simulink model "HMG_1DG1_Test_Cases"  (R2015b)
settings: Solver=ode23tb  StartTime=0.0  StopTime=.3  RelTol=1e-3
undefined symbols (not defined in the file or in its folder): tac, tdc, tdc1
libraries: powerlib x46, powerlib_meascontrol x14, simulink_extras x10, simulink x4
settings Model: Creator=Masoud  LastModifiedBy=Masoud

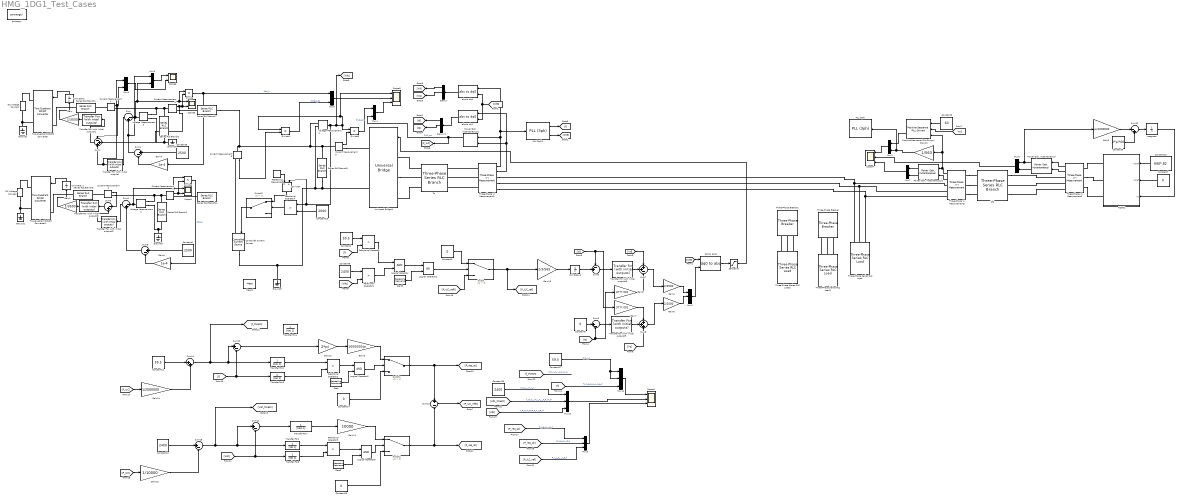
== system HMG_1DG1_Test_Cases ==
  ACDG1 : Subsystem
  Constant1 : Constant  Value=59.5
  Constant10 : Constant  Value=690*.82
  Constant11 : Constant  Value=59.5
  Constant12 : Constant  Value=2400
  Constant{4,6..7,13..14} (5 alike) : Constant  Value=0
  Constant15 : Constant  Value=2000
  Constant16 : Constant  Value=2400
  Constant17 : Constant  Value=59.5
  Constant2 : Constant  Value=2500
  Constant3 : Constant  Value=60
  Constant5 : Constant  Value=2*pi*60
  Constant8 : Constant  Value=2500
  Constant9 : Constant  Value=2400
  Controlled Current Source : powerlib/Electrical Sources/Controlled Current Source  Initialize=on  Source_Type=AC  Amplitude=0  Phase=0  Frequency=0  Measurements=None
  Current Measurement{1..6} (6 alike) : powerlib/Measurements/Current Measurement  PhasorSimulation=off  OutputType=Complex  PSBequivalent=0
  DC Voltage Source1 : powerlib/Electrical Sources/DC Voltage Source  Amplitude=3500  Measurements=None
  DC Voltage Source2 : powerlib/Electrical Sources/DC Voltage Source  Amplitude=3500  Measurements=None
  Demux : Demux  Outputs=3
  Demux1 : Demux  Outputs=3
  Divide{,1..3} (4 alike) : Product  Inputs=**
  Divide4 : Product  Inputs=*/
  Gain : Gain  Gain=1/3500
  Gain1 : Gain  Gain=1/3500
  Gain10 : Gain  Gain=1/563
  Gain11 : Gain  Gain=10000
  Gain12 : Gain  Gain=2*pi
  Gain13 : Gain  Gain=2/3/565
  Gain14 : Gain  Gain=1/2000000
  Gain15 : Gain  Gain=1/10000
  Gain2 : Gain  Gain=2/2500
  Gain3 : Gain  Gain=pi/1000000
  Gain4 : Gain  Gain=1e-4
  Gain5 : Gain  Gain=377*.001
  Gain6 : Gain  Gain=2/2500
  Gain7 : Gain  Gain=377*.001
  Gain8 : Gain  Gain=1e-4
  Gain9 : Gain  Gain=1000000/pi
  Ground{1..5} (5 alike) : powerlib/Elements/Ground  LConnTagsString=a
  Integrator : Integrator
  Logical Operator : Logic  AllPortsSameDT=off  OutDataTypeStr=boolean
  Logical Operator1 : Logic  Operator=OR  AllPortsSameDT=off  OutDataTypeStr=boolean
  Logical Operator2 : Logic  AllPortsSameDT=off  OutDataTypeStr=boolean
  Logical Operator3 : Logic  AllPortsSameDT=off  OutDataTypeStr=boolean
  Mean1 : powerlib_meascontrol/Measurements/Mean  Freq=10  Vinit=0  Ts=0
  Mux{1,4,6..9} (6 alike) : Mux  Inputs=2
  Mux{2..3,5,10..11} (5 alike) : Mux  Inputs=3
  PLL (3ph) : powerlib_meascontrol/PLL/PLL (3ph)  Fmin=45  Par_Init=[0, 60]  ParK=[180, 3200, 1]  TcD=1e-4  MaxRateChangeFreq=12  FilterCutOffFreq=25  Ts=0  AGC=on
  PLL (3ph)1 : powerlib_meascontrol/PLL/PLL (3ph)  Fmin=45  Par_Init=[0, 60]  ParK=[180, 3200, 1]  TcD=1e-4  MaxRateChangeFreq=12  FilterCutOffFreq=25  Ts=0  AGC=on
  Positive-Sequence (PLL-Driven) : powerlib_meascontrol/Measurements/Positive-Sequence (PLL-Driven)  Finit=60  Fmin=45  InInit=[1, 0]  Ts=0
  "Power (3ph, Instantaneous)" : powerlib_meascontrol/Measurements/Power (3ph, Instantaneous)
  "Power (3ph, Instantaneous)1" : powerlib_meascontrol/Measurements/Power (3ph, Instantaneous)
  "Power (3ph, Instantaneous)2" : powerlib_meascontrol/Measurements/Power (3ph, Instantaneous)
  Relational Operator{,1..4} (5 alike) : RelationalOperator  Operator=>  OutDataTypeStr=boolean
  Repeating Sequence3 : simulink/Sources/Repeating Sequence  rep_seq_t=[0 .1 .1001 .2 .2001 10]  rep_seq_y=1e3*[500 500 1800 1800 500 500]
  Saturation : Saturate  UpperLimit=1  LowerLimit=-1
  Scope1 : Scope  NumInputPorts=2
  Scope2 : Scope  NumInputPorts=3
  Scope3 : Scope  NumInputPorts=2
  Scope4 : Scope  NumInputPorts=3
  Scope5 : Scope  NumInputPorts=3
  Scope6 : Scope  NumInputPorts=2
  Series RLC Branch1 : powerlib/Elements/Series RLC Branch  LConnTagsString=__new0  RConnTagsString=__new0  BranchType=RL  Resistance=.05  Inductance=1e-3  SetiL0=off  InitialCurrent=0  Capacitance=1e-6  Setx0=off  InitialVoltage=0  Measurements=None
  Series RLC Branch2 : powerlib/Elements/Series RLC Branch  LConnTagsString=__new0  RConnTagsString=__new0  BranchType=C  Resistance=.05  Inductance=1e-3  SetiL0=off  InitialCurrent=0  Capacitance=4700e-6  Setx0=off  InitialVoltage=0  Measurements=None
  Series RLC Branch3 : powerlib/Elements/Series RLC Branch  LConnTagsString=__new0  RConnTagsString=__new0  BranchType=RL  Resistance=.05  Inductance=1e-3  SetiL0=off  InitialCurrent=0  Capacitance=1e-6  Setx0=off  InitialVoltage=0  Measurements=None
  Series RLC Branch4 : powerlib/Elements/Series RLC Branch  LConnTagsString=__new0  RConnTagsString=__new0  BranchType=C  Resistance=.05  Inductance=1e-3  SetiL0=off  InitialCurrent=0  Capacitance=4700e-6  Setx0=off  InitialVoltage=0  Measurements=None
  Series RLC Branch6 : powerlib/Elements/Series RLC Branch  LConnTagsString=__new0  RConnTagsString=__new0  BranchType=R  Resistance=.01  Inductance=1e-3  SetiL0=off  InitialCurrent=0  Capacitance=1e-6  Setx0=off  InitialVoltage=0  Measurements=None
  Series RLC Branch7 : powerlib/Elements/Series RLC Branch  LConnTagsString=__new0  RConnTagsString=__new0  BranchType=R  Resistance=.01  Inductance=1e-3  SetiL0=off  InitialCurrent=0  Capacitance=1e-6  Setx0=off  InitialVoltage=0  Measurements=None
  Series RLC Branch8 : powerlib/Elements/Series RLC Branch  LConnTagsString=__new0  RConnTagsString=__new0  BranchType=C  Resistance=.05  Inductance=1e-3  SetiL0=off  InitialCurrent=0  Capacitance=4700e-6  Setx0=on  InitialVoltage=2500  Measurements=None
  Start : simulink/Sources/Repeating Sequence  rep_seq_t=[0 .1 .1001 10]  rep_seq_y=[0 0 1 1]
  Start2 : simulink/Sources/Repeating Sequence  rep_seq_t=[0 .1 .1001 10]  rep_seq_y=[0 0 1 1]
  Start3 : simulink/Sources/Repeating Sequence  rep_seq_t=[0 .1 .1001 10]  rep_seq_y=[1 1 0 0]
  Sum{,2..3,12} (4 alike) : Sum  Inputs=|-+
  Sum1 : Sum  Inputs=-++
  Sum{4..5,9..11,15} (6 alike) : Sum  Inputs=|+-
  Sum13 : Sum  Inputs=+-
  Sum14 : Sum  Inputs=|++
  Sum6 : Sum  Inputs=-+|
  Sum7 : Sum  Inputs=++-
  Sum8 : Sum  Inputs=+++
  Switch{,1..3} (4 alike) : Switch  Criteria=u2 > Threshold  Threshold=.5
  Three-Phase Series RLC Load : powerlib/Elements/Three-Phase Series RLC Load  LConnTagsString=A|B|C  Configuration=Y (grounded)  NominalVoltage=690  Vabc=[1e3 1e3 1e3]  Vabcp=[1e3 1e3 1e3]  NominalFrequency=60  UnbalancedPower=off  ActivePower=100e3  InductivePower=0  CapacitivePower=0  Pabc=[10e3 9e3 11e3]  QLabc=[100 90 110]  QCabc=[100 90 110]  Pabcp=[10e3 9e3 11e3]  QLabcp=[100 90 110]  QCabcp=[100 90 110]  Measurements=None  LoadType=constant I
  Three-Phase Series RLC Load1 : powerlib/Elements/Three-Phase Series RLC Load  LConnTagsString=A|B|C  Configuration=Y (grounded)  NominalVoltage=690  Vabc=[1e3 1e3 1e3]  Vabcp=[1e3 1e3 1e3]  NominalFrequency=60  UnbalancedPower=off  ActivePower=1200e3  InductivePower=0  CapacitivePower=0  Pabc=[10e3 9e3 11e3]  QLabc=[100 90 110]  QCabc=[100 90 110]  Pabcp=[10e3 9e3 11e3]  QLabcp=[100 90 110]  QCabcp=[100 90 110]  Measurements=None  LoadType=constant I
  Three-Phase Series RLC Load2 : powerlib/Elements/Three-Phase Series RLC Load  LConnTagsString=A|B|C  Configuration=Y (grounded)  NominalVoltage=690  Vabc=[1e3 1e3 1e3]  Vabcp=[1e3 1e3 1e3]  NominalFrequency=60  UnbalancedPower=off  ActivePower=500e3  InductivePower=0  CapacitivePower=0  Pabc=[10e3 9e3 11e3]  QLabc=[100 90 110]  QCabc=[100 90 110]  Pabcp=[10e3 9e3 11e3]  QLabcp=[100 90 110]  QCabcp=[100 90 110]  Measurements=None  LoadType=constant I
  Three-Phase V-I Measurement1 : powerlib/Measurements/Three-Phase V-I Measurement  VoltageMeasurement=phase-to-ground  SetLabelV=off  LabelV=Vabc  Vpu=off  VpuLL=off  CurrentMeasurement=yes  SetLabelI=off  LabelI=Iabc  Ipu=off  Pbase=100e6  Vbase=500e3  OutputType=Complex  PhasorSimulation=off  PSBequivalent=0
  Three-Phase V-I Measurement2 : powerlib/Measurements/Three-Phase V-I Measurement  VoltageMeasurement=phase-to-ground  SetLabelV=off  LabelV=Vabc  Vpu=off  VpuLL=off  CurrentMeasurement=yes  SetLabelI=off  LabelI=Iabc  Ipu=off  Pbase=100e6  Vbase=500e3  OutputType=Complex  PhasorSimulation=off  PSBequivalent=0
  Three-Phase V-I Measurement5 : powerlib/Measurements/Three-Phase V-I Measurement  VoltageMeasurement=phase-to-ground  SetLabelV=off  LabelV=Vabc  Vpu=off  VpuLL=off  CurrentMeasurement=yes  SetLabelI=off  LabelI=Iabc  Ipu=off  Pbase=100e6  Vbase=500e3  OutputType=Complex  PhasorSimulation=off  PSBequivalent=0
  Three-Phase Breaker : powerlib/Elements/Three-Phase Breaker  InitialState=open  SwitchA=on  SwitchB=on  SwitchC=on  SwitchTimes=[.2 .6]  External=off  BreakerResistance=0.01  SnubberResistance=1e6  SnubberCapacitance=inf  Measurements=None
  Three-Phase Breaker1 : powerlib/Elements/Three-Phase Breaker  InitialState=open  SwitchA=on  SwitchB=on  SwitchC=on  SwitchTimes=[.4 .7]  External=off  BreakerResistance=0.01  SnubberResistance=1e6  SnubberCapacitance=inf  Measurements=None
  Transfer Fcn (with initial outputs) : simulink_extras/Additional Linear/Transfer Fcn (with initial outputs)  N=[8 1]  D=[1 0]  Y0=.5  U0=0
  Transfer Fcn (with initial outputs)1 : simulink_extras/Additional Linear/Transfer Fcn (with initial outputs)  N=[2.5 250]  D=[1 0]  Y0=.5  U0=0
  Transfer Fcn (with initial outputs)2 : simulink_extras/Additional Linear/Transfer Fcn (with initial outputs)  N=[4 19.2]  D=[1 0]  Y0=.5  U0=0
  Transfer Fcn (with initial outputs)3 : simulink_extras/Additional Linear/Transfer Fcn (with initial outputs)  N=[2.5 250]  D=[1 0]  Y0=.5  U0=0
  Transfer Fcn (with initial outputs)5 : simulink_extras/Additional Linear/Transfer Fcn (with initial outputs)  N=[10.5 175]  D=[1 0]  Y0=.5  U0=0
  Transfer Fcn (with initial outputs)6 : simulink_extras/Additional Linear/Transfer Fcn (with initial outputs)  N=[10.5 175]  D=[1 0]  Y0=.5  U0=0
  Transfer Fcn1 : TransferFcn  Denominator=[tdc 1]
  Transfer Fcn2 : TransferFcn  Denominator=[tac 1]
  Transfer Fcn3 : TransferFcn  Denominator=[tac 1]
  Transfer Fcn4 : TransferFcn  Denominator=[tac 1]
  Transfer Fcn7 : TransferFcn  Denominator=[tdc1 1]
  Transfer Fcn8 : TransferFcn  Denominator=[tdc 1]
  Two-Quadrant DC/DC Converter : powerlib/Power Electronics/Two-Quadrant DC//DC Converter  ModelType=Average model (D-controlled)  Ron=1e-3  Rs=1e6  Cs=inf  Vforward=[ 0, 0 ]  Ron_Diode=1e-3  Rs_Diode=1e6  Cs_Diode=inf  Vf_Diode=1e-3  Rs_CurrentSource=inf
      settings: AttributesFormatString=%<ModelType>
  Two-Quadrant DC/DC Converter1 : powerlib/Power Electronics/Two-Quadrant DC//DC Converter  ModelType=Average model (D-controlled)  Ron=1e-3  Rs=1e6  Cs=inf  Vforward=[ 0, 0 ]  Ron_Diode=1e-3  Rs_Diode=1e6  Cs_Diode=inf  Vf_Diode=1e-3  Rs_CurrentSource=inf
      settings: AttributesFormatString=%<ModelType>
  Unit Delay : UnitDelay  SampleTime=5e-5
  Unit Delay1 : UnitDelay  SampleTime=5e-5
  Unit Delay2 : UnitDelay  SampleTime=5e-5
  Universal Bridge1 : powerlib/Power Electronics/Universal Bridge  Arms=3  SnubberResistance=1e5  SnubberCapacitance=inf  Device=Average-model based VSC  Ron=1e-3  Lon=0  ForwardVoltages="[  0  0  ]"  ForwardVoltage=0  GTOparameters=[ 10e-6 , 20e-6 ]  IGBTparameters=[ 1e-6 , 2e-6 ]  Measurements=None  Measurements_2=None  converterType=Rectifier
  Voltage Measurement1 : powerlib/Measurements/Voltage Measurement  PhasorSimulation=off  OutputType=Complex  PSBequivalent=0
  Voltage Measurement2 : powerlib/Measurements/Voltage Measurement  PhasorSimulation=off  OutputType=Complex  PSBequivalent=0
  Voltage Measurement3 : powerlib/Measurements/Voltage Measurement  PhasorSimulation=off  OutputType=Complex  PSBequivalent=0
  Zc : powerlib/Elements/Three-Phase Series RLC Branch  LConnTagsString=A|B|C  RConnTagsString=A|B|C  BranchType=RL  Resistance=.01  Inductance=1e-3  Capacitance=1e-6  Measurements=None
  Zc2 : powerlib/Elements/Three-Phase Series RLC Branch  LConnTagsString=A|B|C  RConnTagsString=A|B|C  BranchType=RL  Resistance=.0001  Inductance=1e-5  Capacitance=1e-6  Measurements=None
  abc to dq0 : powerlib_meascontrol/Transformations/abc to dq0  Alignment=90 degrees behind phase A axis
  abc to dq1 : powerlib_meascontrol/Transformations/abc to dq0  Alignment=90 degrees behind phase A axis
  dq0 to abc1 : powerlib_meascontrol/Transformations/dq0 to abc  Alignment=90 degrees behind phase A axis
  powergui : powerlib/powergui  Priority=2  SimulationMode=Discrete  SolverType=Tustin  SampleTime=10e-5  frequency=60  SPID=off  DisableSnubberDevices=off  DisableRonSwitches=off  DisableVfSwitches=off  SwTol=0  DisplayEquations=off  Interpol=off  ExternalGateDelay=off  methode=off  Ts=0  FunctionMessages=off  echomessages=off  HookPort=off  EnableUseOfTLC=off  x0status=blocks  frequencyindice=0  Pbase=100e6  ErrMax=1e-4  Iterations=50  UnitsV=kV  UnitsW=MW  buscounter=0  RestoreLinks=warning  ResistiveCurrentMeasurement=off  Frange=[0:2:500]  Ylog=off  Xlog=on  ShowGrid=off  save=off  variable=ZData  structure=inserted_I  ZoomFFT=off  StartTime=0.15  cycles=50  DisplayStyle=4  fundamental=600  FreqAxis=off  MaxFrequency=700  frequencyindicesteady=1  RmsSteady=1  display=off
  wires:
  Voltage Measurement3/1 -> Mux8/2, Scope3/1, Divide/1, Sum/1
  Sum4/1 -> Mux8/1, Sum/2
  Sum/1 -> Transfer Fcn (with initial outputs)/1
  Current Measurement1/1 -> Sum1/1, Mux9/2
  Sum1/1 -> Transfer Fcn (with initial outputs)1/1
  Gain/1 -> Unit Delay/1
  Unit Delay/1 -> Two-Quadrant DC/DC Converter/1
  Transfer Fcn (with initial outputs)1/1 -> Gain/1
  Current Measurement4/1 -> Sum1/2, Scope3/2, Divide/2
  Voltage Measurement1/1 -> Sum2/1, Divide2/1, Scope1/1
  Sum2/1 -> Transfer Fcn (with initial outputs)2/1
  Transfer Fcn (with initial outputs)2/1 -> Sum3/2
  Current Measurement2/1 -> Sum3/1
  Sum3/1 -> Transfer Fcn (with initial outputs)3/1
  Gain1/1 -> Unit Delay1/1
  Unit Delay1/1 -> Two-Quadrant DC/DC Converter1/1
  Transfer Fcn (with initial outputs)3/1 -> Gain1/1
  Current Measurement3/1 -> Divide2/2, Scope1/2
  Constant5/1 -> Sum12/2
  Integrator/1 -> ACDG1/3(wt)
  Three-Phase V-I Measurement2/2 -> "Power (3ph, Instantaneous)"/2
  Three-Phase V-I Measurement2/1 -> "Power (3ph, Instantaneous)"/1
  "Power (3ph, Instantaneous)"/2 -> Mux6/2
  Three-Phase V-I Measurement5/1 -> Positive-Sequence (PLL-Driven)/3, Gain10/1, "Power (3ph, Instantaneous)1"/1
  Three-Phase V-I Measurement5/2 -> "Power (3ph, Instantaneous)1"/2
  "Power (3ph, Instantaneous)1"/1 -> Mux7/1
  "Power (3ph, Instantaneous)1"/2 -> Mux7/2
  "Power (3ph, Instantaneous)"/1 -> Gain3/1, Mux6/1
  Gain3/1 -> Sum12/1
  Sum12/1 -> Integrator/1
  [wt1] -> Positive-Sequence (PLL-Driven)/2
  Constant3/1 -> Positive-Sequence (PLL-Driven)/1
  Constant10/1 -> ACDG1/1(Vdref)
  Constant7/1 -> ACDG1/2(Vqref)
  Positive-Sequence (PLL-Driven)/2 -> Mux1/1
  Gain10/1 -> PLL (3ph)/1, Mux1/2
  Mux1/1 -> Scope4/1
  Mux6/1 -> Scope4/2
  Mux7/1 -> Scope4/3
  Sum5/1 -> Transfer Fcn (with initial outputs)5/1
  Sum6/1 -> Transfer Fcn (with initial outputs)6/1
  Mux2/1 -> dq0 to abc1/1
  dq0 to abc1/1 -> Saturation/1
  Saturation/1 -> Universal Bridge1/1
  Transfer Fcn (with initial outputs)6/1 -> Sum7/2
  Gain5/1 -> Sum7/3
  Sum7/1 -> Gain2/1
  Transfer Fcn (with initial outputs)5/1 -> Sum8/2
  Sum8/1 -> Gain6/1
  [wt3] -> dq0 to abc1/2
  [Vd] -> Sum7/1
  Gain2/1 -> Mux2/1
  Gain6/1 -> Mux2/2
  [Vq] -> Sum8/3
  Gain7/1 -> Sum8/1
  [Id] -> Gain7/1, Sum6/1
  [Iq] -> Gain5/1, Sum5/2
  Constant6/1 -> Sum5/1
  Three-Phase V-I Measurement1/2 -> "Power (3ph, Instantaneous)2"/2, abc to dq1/1
  Three-Phase V-I Measurement1/1 -> "Power (3ph, Instantaneous)2"/1, PLL (3ph)1/1, abc to dq0/1
  abc to dq1/1 -> Demux1/1
  abc to dq0/1 -> Demux/1
  [wt3] -> abc to dq1/2, abc to dq0/2
  Demux1/1 -> [Id]
  Demux1/2 -> [Iq]
  Demux/1 -> [Vd]
  Demux/2 -> [Vq]
  PLL (3ph)1/2 -> [wt3]
  Constant8/1 -> Sum4/1
  Divide/1 -> Mux3/1, Gain4/1  "Pdc_1"
  Gain4/1 -> Sum4/2
  Voltage Measurement2/1 -> Divide4/2, Relational Operator4/1, [Vdc], Divide3/1, Scope5/1, Divide1/1
  Current Measurement6/1 -> Divide1/2
  Sum9/1 -> Sum2/2
  Constant2/1 -> Sum9/1
  Divide2/1 -> Gain8/1  "Pdc_2"
  Gain8/1 -> Sum9/2
  Divide1/1 -> Mux3/3  "Pload_dc"
  Mux3/1 -> Scope5/2
  Current Measurement5/1 -> Divide3/2
  Divide3/1 -> Mux4/1  "PILC_dc"
  "Power (3ph, Instantaneous)2"/1 -> [P_ILC], Mux4/2  "PILC_ac"
  Mux4/1 -> Scope5/3
  PLL (3ph)1/1 -> [f]
  [f] -> Relational Operator/2
  Constant1/1 -> Relational Operator/1
  Relational Operator/1 -> Logical Operator/1
  Constant9/1 -> Relational Operator1/1
  [Vdc] -> Relational Operator1/2
  Relational Operator1/1 -> Logical Operator/2
  Logical Operator/1 -> Logical Operator1/1
  Constant4/1 -> Switch/1
  [f] -> Transfer Fcn3/1, Sum10/2
  Sum14/1 -> [f_thresh], Transfer Fcn2/1, Sum10/1
  Relational Operator2/1 -> Logical Operator2/1
  Constant14/1 -> Switch1/3
  Gain9/1 -> Switch1/1
  Constant13/1 -> Switch2/3
  Gain11/1 -> Switch2/1
  Switch2/1 -> [P_req_dc], Sum13/2
  Switch1/1 -> [P_req_ac], Sum13/1
  Sum13/1 -> [P_ILC_ref0]
  Switch/1 -> [P_ILC_ref], Gain13/1
  Mux5/1 -> Scope2/3
  Start3/1 -> Logical Operator1/2
  Logical Operator1/1 -> Switch/2
  Start/1 -> Logical Operator2/2
  Logical Operator2/1 -> Switch1/2
  Logical Operator3/1 -> Switch2/2
  Start2/1 -> Logical Operator3/2
  Relational Operator3/1 -> Logical Operator3/1
  Gain12/1 -> Gain9/1
  Unit Delay2/1 -> Sum6/2
  Constant11/1 -> Sum14/1
  [P_ILC] -> Gain14/1
  Transfer Fcn2/1 -> Relational Operator2/1
  Transfer Fcn3/1 -> Relational Operator2/2
  Constant12/1 -> Sum15/1
  [P_ILC] -> Gain15/1
  Sum15/1 -> [Vdc_thresh], Transfer Fcn1/1, Sum11/1
  [Vdc] -> Sum11/2, Transfer Fcn8/1
  Constant15/1 -> Relational Operator4/2
  Relational Operator4/1 -> Switch3/2
  Repeating Sequence3/1 -> Divide4/1
  Divide4/1 -> Switch3/1
  Mux8/1 -> Scope6/1
  Mux9/1 -> Scope6/2
  Transfer Fcn (with initial outputs)/1 -> Sum1/3, Mux9/1
  Gain13/1 -> Unit Delay2/1
  [P_ILC_ref0] -> Switch/3
  [P_req_ac] -> Mux5/1  "P_r_e_q_,_a_c"
  [P_req_dc] -> Mux5/2  "P_r_e_q_,_d_c"
  Mux11/1 -> Scope2/1
  [P_ILC_ref] -> Mux5/3  "P_I_L_C_,_r_e_f"
  Constant17/1 -> Mux11/2, Mux11/1  "f_m_i_n"
  [f] -> Mux11/3  "f_m_e_a_s_u_r_e_d"
  Mux10/1 -> Scope2/2
  Constant16/1 -> Mux10/1  "V_d_c_,_m_i_n"
  [Vdc] -> Mux10/3  "V_d_c_m_e_a_s_u_r_e_d"
  [Vdc_thresh] -> Mux10/2  "V_d_c_,_m_i_n_,_c_o_m_p"
  [f_thresh] -> ?  "f_m_i_n_,_c_o_m_p"
  Sum10/1 -> Gain12/1
  Sum11/1 -> Transfer Fcn7/1
  Switch3/1 -> Controlled Current Source/1
  Gain15/1 -> Sum15/2
  Gain14/1 -> Sum14/2
  Transfer Fcn7/1 -> Gain11/1
  Transfer Fcn1/1 -> Relational Operator3/1
  Transfer Fcn8/1 -> Relational Operator3/2
  connections:
  DC Voltage Source1/LConn1 -- Ground1/LConn1 -- Two-Quadrant DC/DC Converter/RConn2
  Two-Quadrant DC/DC Converter/RConn1 -- DC Voltage Source1/RConn1
  Two-Quadrant DC/DC Converter/LConn1 -- Series RLC Branch1/LConn1
  Series RLC Branch2/LConn1 -- Voltage Measurement3/LConn1 -- Current Measurement1/RConn1 -- Current Measurement4/LConn1
  Current Measurement1/LConn1 -- Series RLC Branch1/RConn1
  Ground4/LConn1 -- Voltage Measurement3/LConn2 -- Series RLC Branch2/RConn1
  DC Voltage Source2/LConn1 -- Two-Quadrant DC/DC Converter1/RConn2 -- Ground2/LConn1
  Series RLC Branch4/LConn1 -- Current Measurement3/LConn1 -- Current Measurement2/RConn1 -- Voltage Measurement1/LConn1
  Series RLC Branch4/RConn1 -- Voltage Measurement1/LConn2 -- Ground5/LConn1
  Two-Quadrant DC/DC Converter1/LConn1 -- Series RLC Branch3/LConn1
  Two-Quadrant DC/DC Converter1/RConn1 -- DC Voltage Source2/RConn1
  Current Measurement2/LConn1 -- Series RLC Branch3/RConn1
  Series RLC Branch6/LConn1 -- Current Measurement3/RConn1
  Current Measurement4/RConn1 -- Series RLC Branch7/LConn1
  Zc2/RConn1 -- Three-Phase V-I Measurement2/RConn1
  Three-Phase V-I Measurement2/RConn2 -- Zc2/RConn2
  Zc2/RConn3 -- Three-Phase V-I Measurement2/RConn3
  Three-Phase V-I Measurement5/LConn1 -- Zc2/LConn1
  Three-Phase V-I Measurement5/LConn2 -- Zc2/LConn2
  Three-Phase V-I Measurement5/LConn3 -- Zc2/LConn3
  Three-Phase V-I Measurement5/RConn1 -- Three-Phase V-I Measurement1/RConn1 -- Three-Phase Series RLC Load/LConn1
  Three-Phase V-I Measurement5/RConn2 -- Three-Phase V-I Measurement1/RConn2 -- Three-Phase Series RLC Load/LConn2
  Three-Phase V-I Measurement5/RConn3 -- Three-Phase V-I Measurement1/RConn3 -- Three-Phase Series RLC Load/LConn3
  Three-Phase Series RLC Load1/LConn1 -- Three-Phase Breaker/RConn1
  Three-Phase Series RLC Load1/LConn2 -- Three-Phase Breaker/RConn2
  Three-Phase Series RLC Load1/LConn3 -- Three-Phase Breaker/RConn3
  Three-Phase V-I Measurement2/LConn1 -- ACDG1/RConn1
  Three-Phase V-I Measurement2/LConn2 -- ACDG1/RConn2
  Three-Phase V-I Measurement2/LConn3 -- ACDG1/RConn3
  Zc/LConn1 -- Universal Bridge1/LConn1
  Universal Bridge1/LConn2 -- Zc/LConn2
  Zc/LConn3 -- Universal Bridge1/LConn3
  Three-Phase V-I Measurement1/LConn1 -- Zc/RConn1
  Three-Phase V-I Measurement1/LConn2 -- Zc/RConn2
  Three-Phase V-I Measurement1/LConn3 -- Zc/RConn3
  Current Measurement5/RConn1 -- Universal Bridge1/RConn1
  Ground3/LConn1 -- Series RLC Branch8/RConn1 -- Universal Bridge1/RConn2 -- Voltage Measurement2/LConn2 -- Controlled Current Source/RConn1
  Series RLC Branch7/RConn1 -- Current Measurement6/LConn1 -- Series RLC Branch8/LConn1 -- Current Measurement5/LConn1 -- Voltage Measurement2/LConn1
  Controlled Current Source/LConn1 -- Current Measurement6/RConn1
  Three-Phase Series RLC Load2/LConn3 -- Three-Phase Breaker1/RConn3
  Three-Phase Series RLC Load2/LConn2 -- Three-Phase Breaker1/RConn2
  Three-Phase Series RLC Load2/LConn1 -- Three-Phase Breaker1/RConn1

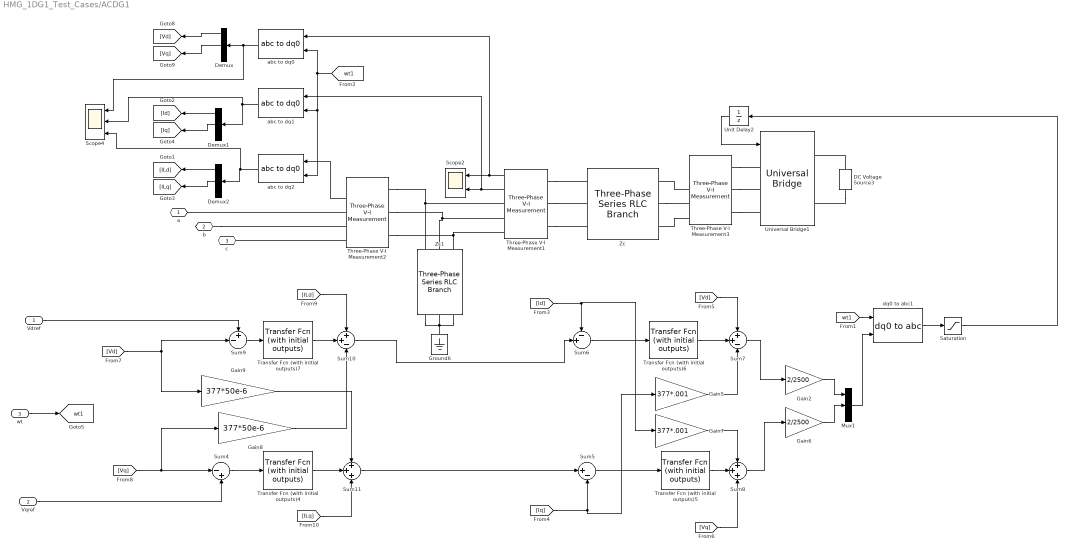
== system HMG_1DG1_Test_Cases/ACDG1 ==
  Vdref : Inport
  Vqref : Inport  Port=2
  wt : Inport  Port=3
  DC Voltage Source3 : powerlib/Electrical Sources/DC Voltage Source  Amplitude=2500  Measurements=None
  Demux : Demux  Outputs=3
  Demux1 : Demux  Outputs=3
  Demux2 : Demux  Outputs=3
  Gain2 : Gain  Gain=2/2500
  Gain5 : Gain  Gain=377*.001
  Gain6 : Gain  Gain=2/2500
  Gain7 : Gain  Gain=377*.001
  Gain8 : Gain  Gain=377*50e-6
  Gain9 : Gain  Gain=377*50e-6
  Ground6 : powerlib/Elements/Ground  LConnTagsString=a
  Mux1 : Mux  Inputs=3
  Saturation : Saturate  UpperLimit=1  LowerLimit=-1
  Scope2 : Scope  NumInputPorts=2
  Scope4 : Scope  NumInputPorts=3
  Sum10 : Sum  Inputs=++-
  Sum11 : Sum  Inputs=+++
  Sum4 : Sum  Inputs=|-+
  Sum5 : Sum  Inputs=|+-
  Sum6 : Sum  Inputs=-+|
  Sum7 : Sum  Inputs=++-
  Sum8 : Sum  Inputs=+++
  Sum9 : Sum  Inputs=+-|
  Three-Phase V-I Measurement1 : powerlib/Measurements/Three-Phase V-I Measurement  VoltageMeasurement=phase-to-ground  SetLabelV=off  LabelV=Vabc  Vpu=off  VpuLL=off  CurrentMeasurement=yes  SetLabelI=off  LabelI=Iabc  Ipu=off  Pbase=100e6  Vbase=500e3  OutputType=Complex  PhasorSimulation=off  PSBequivalent=0
  Three-Phase V-I Measurement2 : powerlib/Measurements/Three-Phase V-I Measurement  VoltageMeasurement=phase-to-ground  SetLabelV=off  LabelV=Vabc  Vpu=off  VpuLL=off  CurrentMeasurement=yes  SetLabelI=off  LabelI=Iabc  Ipu=off  Pbase=100e6  Vbase=500e3  OutputType=Complex  PhasorSimulation=off  PSBequivalent=0
  Three-Phase V-I Measurement3 : powerlib/Measurements/Three-Phase V-I Measurement  VoltageMeasurement=phase-to-ground  SetLabelV=off  LabelV=Vabc  Vpu=off  VpuLL=off  CurrentMeasurement=yes  SetLabelI=off  LabelI=Iabc  Ipu=off  Pbase=100e6  Vbase=500e3  OutputType=Complex  PhasorSimulation=off  PSBequivalent=0
  Transfer Fcn (with initial outputs)4 : simulink_extras/Additional Linear/Transfer Fcn (with initial outputs)  N=[.1 50]  D=[1 0]  Y0=.5  U0=0
  Transfer Fcn (with initial outputs)5 : simulink_extras/Additional Linear/Transfer Fcn (with initial outputs)  N=[10.5 175]  D=[1 0]  Y0=.5  U0=0
  Transfer Fcn (with initial outputs)6 : simulink_extras/Additional Linear/Transfer Fcn (with initial outputs)  N=[10.5 175]  D=[1 0]  Y0=.5  U0=0
  Transfer Fcn (with initial outputs)7 : simulink_extras/Additional Linear/Transfer Fcn (with initial outputs)  N=[.1 50]  D=[1 0]  Y0=.5  U0=0
  Unit Delay2 : UnitDelay  SampleTime=5e-5
  Universal Bridge1 : powerlib/Power Electronics/Universal Bridge  Arms=3  SnubberResistance=1e5  SnubberCapacitance=inf  Device=Average-model based VSC  Ron=1e-3  Lon=0  ForwardVoltages="[  0  0  ]"  ForwardVoltage=0  GTOparameters=[ 10e-6 , 20e-6 ]  IGBTparameters=[ 1e-6 , 2e-6 ]  Measurements=None  Measurements_2=None  converterType=Rectifier
  Zc : powerlib/Elements/Three-Phase Series RLC Branch  LConnTagsString=A|B|C  RConnTagsString=A|B|C  BranchType=RL  Resistance=.01  Inductance=1e-3  Capacitance=1e-6  Measurements=None
  Zc1 : powerlib/Elements/Three-Phase Series RLC Branch  LConnTagsString=A|B|C  RConnTagsString=A|B|C  BranchType=C  Resistance=.01  Inductance=1e-3  Capacitance=50e-6  Measurements=None
  abc to dq0 : powerlib_meascontrol/Transformations/abc to dq0  Alignment=90 degrees behind phase A axis
  abc to dq1 : powerlib_meascontrol/Transformations/abc to dq0  Alignment=90 degrees behind phase A axis
  abc to dq2 : powerlib_meascontrol/Transformations/abc to dq0  Alignment=90 degrees behind phase A axis
  dq0 to abc1 : powerlib_meascontrol/Transformations/dq0 to abc  Alignment=90 degrees behind phase A axis
  a : PMIOPort  Port=1  Side=Right
  b : PMIOPort  Port=2  Side=Right
  c : PMIOPort  Port=3  Side=Right
  tag scope: wt1=global
  wires:
  Sum4/1 -> Transfer Fcn (with initial outputs)4/1
  Three-Phase V-I Measurement1/2 -> abc to dq1/1, Scope2/2
  Sum5/1 -> Transfer Fcn (with initial outputs)5/1
  Sum6/1 -> Transfer Fcn (with initial outputs)6/1
  Mux1/1 -> dq0 to abc1/1
  dq0 to abc1/1 -> Saturation/1
  Saturation/1 -> Unit Delay2/1
  Unit Delay2/1 -> Universal Bridge1/1
  Transfer Fcn (with initial outputs)6/1 -> Sum7/2
  Gain5/1 -> Sum7/3
  Sum7/1 -> Gain2/1
  Transfer Fcn (with initial outputs)5/1 -> Sum8/2
  Sum8/1 -> Gain6/1
  Three-Phase V-I Measurement1/1 -> abc to dq0/1, Scope2/1
  [wt1] -> dq0 to abc1/2
  Vqref/1 -> Sum4/2
  [Vd] -> Sum7/1
  Sum9/1 -> Transfer Fcn (with initial outputs)7/1
  Transfer Fcn (with initial outputs)7/1 -> Sum10/2
  [ILd] -> Sum10/1
  [ILq] -> Sum11/3
  Transfer Fcn (with initial outputs)4/1 -> Sum11/2
  Gain8/1 -> Sum10/3
  Gain9/1 -> Sum11/1
  Gain2/1 -> Mux1/1
  Gain6/1 -> Mux1/2
  [Vq] -> Gain8/1, Sum4/1
  [Vd] -> Sum9/2, Gain9/1
  Vdref/1 -> Sum9/1
  abc to dq1/1 -> Scope4/2, Demux1/1
  abc to dq0/1 -> Scope4/1, Demux/1
  [wt1] -> abc to dq2/2, abc to dq1/2, abc to dq0/2
  Demux1/1 -> [Id]
  Demux1/2 -> [Iq]
  Demux/1 -> [Vd]
  Demux/2 -> [Vq]
  Three-Phase V-I Measurement2/2 -> abc to dq2/1
  abc to dq2/1 -> Scope4/3, Demux2/1
  Demux2/1 -> [ILd]
  Demux2/2 -> [ILq]
  [Vq] -> Sum8/3
  Gain7/1 -> Sum8/1
  [Id] -> Gain7/1, Sum6/1
  [Iq] -> Gain5/1, Sum5/2
  Sum10/1 -> Sum6/2
  Sum11/1 -> Sum5/1
  wt/1 -> [wt1]
  connections:
  Three-Phase V-I Measurement1/RConn1 -- Three-Phase V-I Measurement2/LConn1 -- Zc1/LConn1
  Three-Phase V-I Measurement1/RConn2 -- Three-Phase V-I Measurement2/LConn2 -- Zc1/LConn2
  Zc1/RConn1 -- Zc1/RConn2 -- Ground6/LConn1 -- Zc1/RConn3
  Three-Phase V-I Measurement1/RConn3 -- Zc1/LConn3 -- Three-Phase V-I Measurement2/LConn3
  DC Voltage Source3/RConn1 -- Universal Bridge1/RConn1
  Three-Phase V-I Measurement1/LConn1 -- Zc/LConn1
  DC Voltage Source3/LConn1 -- Universal Bridge1/RConn2
  Three-Phase V-I Measurement3/RConn1 -- Zc/RConn1
  Three-Phase V-I Measurement3/LConn3 -- Universal Bridge1/LConn3
  Three-Phase V-I Measurement3/LConn1 -- Universal Bridge1/LConn1
  Three-Phase V-I Measurement1/LConn3 -- Zc/LConn3
  Three-Phase V-I Measurement1/LConn2 -- Zc/LConn2
  Zc/RConn2 -- Three-Phase V-I Measurement3/RConn2
  Three-Phase V-I Measurement3/LConn2 -- Universal Bridge1/LConn2
  Three-Phase V-I Measurement3/RConn3 -- Zc/RConn3
  Three-Phase V-I Measurement2/RConn1 -- a/RConn1
  b/RConn1 -- Three-Phase V-I Measurement2/RConn2
  Three-Phase V-I Measurement2/RConn3 -- c/RConn1
